simulink model "TST_StateflowDefaultTransitionCondition"  (Simulink 7.4)
settings: Solver=FixedStepDiscrete  StartTime=0.0  StopTime=10.0  FixedStep=0.02  RelTol=1e-3
settings Model: Creator=kharthforeign  LastModifiedBy=kharthforeign  BufferReuse=off
settings DataIOCC: SaveOutput=off  SignalLogging=off  SaveTime=off
settings OptimizationCC: BlockReduction=off  ConditionallyExecuteInputs=off  OptimizeBlockIOStorage=off  BufferReuse=off  ExpressionFolding=off  LocalBlockOutputs=off  InitFltsAndDblsToZero=on

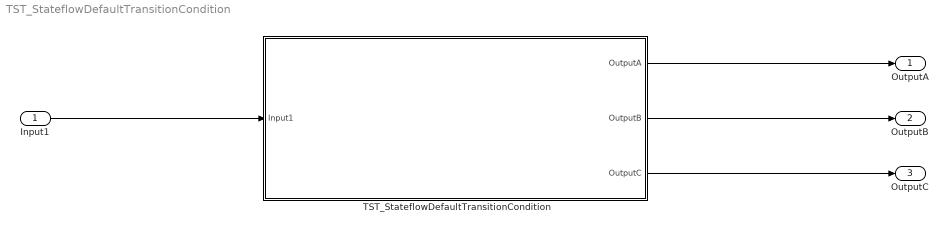
== system TST_StateflowDefaultTransitionCondition ==
  Input1 : Inport  DataType=uint32  OutDataType=fixdt(1, 16)  OutScaling=2^0  OutDataTypeStr=uint32  BusOutputAsStruct=on
  TST_StateflowDefaultTransitionCondition : Subsystem  TreatAsAtomicUnit=on
  OutputA : Outport  PortDimensions=1  DataType=double  OutDataType=fixdt(1, 16)  OutScaling=2^0  OutDataTypeStr=double
  OutputB : Outport  Port=2  PortDimensions=1  DataType=double  OutDataType=Enum: DIL_VmmGsFcsCommandsMessage_LatApModeCmd  OutDataTypeStr=double
  OutputC : Outport  Port=3  PortDimensions=1  DataType=double  OutDataType=fixdt(1, 16)  OutScaling=2^0  OutDataTypeStr=double
  wires:
  Input1/1 -> TST_StateflowDefaultTransitionCondition/1(Input1)
  TST_StateflowDefaultTransitionCondition/1(OutputA) -> OutputA/1
  TST_StateflowDefaultTransitionCondition/2(OutputB) -> OutputB/1
  TST_StateflowDefaultTransitionCondition/3(OutputC) -> OutputC/1

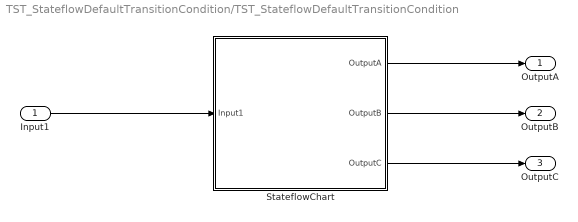
== system TST_StateflowDefaultTransitionCondition/TST_StateflowDefaultTransitionCondition ==
  Input1 : Inport  DataType=uint32  OutDataType=fixdt(1, 16)  OutScaling=2^0  OutDataTypeStr=uint32  BusOutputAsStruct=on
  StateflowChart : Stateflow chart
  OutputA : Outport  PortDimensions=1  DataType=double  OutDataType=fixdt(1, 16)  OutScaling=2^0  OutDataTypeStr=double
  OutputB : Outport  Port=2  PortDimensions=1  DataType=double  OutDataType=Enum: DIL_VmmGsFcsCommandsMessage_LatApModeCmd  OutDataTypeStr=double
  OutputC : Outport  Port=3  PortDimensions=1  DataType=double  OutDataType=fixdt(1, 16)  OutScaling=2^0  OutDataTypeStr=double
  wires:
  StateflowChart/1(OutputA) -> OutputA/1
  StateflowChart/2(OutputB) -> OutputB/1
  StateflowChart/3(OutputC) -> OutputC/1
  Input1/1 -> StateflowChart/1(Input1)

== stateflow chart TST_StateflowDefaultTransitionCondition/StateflowChart ==
  state StateA
    entry:
    OutputA = 10.0;
  state StateB
    entry:
    OutputB = 20.0;
    state Ping
    state Pong
    (default) -> Ping
    Ping -> Pong : [A]
    Pong -> Ping : [B]
  state ResultA = EvaluateConditionA(X) [function]
    (default) -> (junction 9) : [X > 123.0]...
        | {ResultA = false;}
  state ResultB = EvaluateConditionB(X) [function]
    (default) -> (junction 10)
    (junction 10) -> (junction 11) : [X > 123.0]...
        | {ResultB = false;}
  StateA -> StateB : [EvaluateConditionB(Local)]
  StateB -> StateA : [EvaluateConditionA(-1.0 * Local)]
  (default) -> StateA : [A && B]...
      | {Local = 5.0;}
  data: X function_input double; ResultA function_output boolean =true; X function_input double; ResultB function_output boolean =true; Input1 input uint32; OutputA output double =1; OutputB output double =2; OutputC output double =3; Local local double =0; A local boolean; B local boolean; C local boolean
